simulink model "vehicle_hostmodel_2022b_v10"  (R2024b)
settings: Solver=ode4  StartTime=0.0  StopTime=inf  FixedStep=0.01  MaxStep=0.05  RelTol=1e-3
PreLoadFcn:
  | load("FInalGraph.mat")
model workspace (MAT data in the model file):
  G_final : digraph (value not decoded)
values from neighbouring files (symbols this model uses):
  ActorID = 0    [HelperSpeedActionAdapter.m]
  D = cross(B-A,C-A)    [HelperCalculateEgoRefPathInfo.m]
  L = zeros(N,1)    [HelperCalculateEgoRefPathInfo.m]
  psi_o = -1.185    [sensor.m]
  R = NaN(N,1)    [HelperCalculateEgoRefPathInfo.m]
  SceneInfo = [-32.1351766513 25.1612903226 -74.2242703533 -71.4592933948 -32.2887864823 26.2365591398 26.8509984639 27.0046082949 -32.7496159754 -72.380952381 -49.846390169 -49.3855606759 ... (30 elements, 10x3)]    [SceneLabels.mat]
  Ts = 0.05    [sensor.m]
undefined symbols (not defined in the file or in its folder): Acceleration, AngularVelocity, barrier_1, barrier_2, barrier_3, curvature, DefaultGear, DEND_B, DEND_S, DEND_T, direction, DiscIntNeverNeededParam, driving, finalint, goal1_coordinates, goal2_coordinates, goal3_coordinates, gradbp, latlongcoordinates, LF, LR, matlabshared, MAX_BRAKE, MAX_STEER, MAX_TORQUE, MCAR, MIN_BRAKE, MIN_STEER, MIN_TORQUE, NUMD_B, NUMD_S, NUMD_T, Pitch, Position, Roll, RRdamp, session, sigbuilder_block, STEER_RATIO, stopSign_ID, Tdead, thetaRefs, TL_ID, TrackWidth, ts, Vdead, Velocity, WB, xRef2s, Yaw, yRef2s
libraries: simulink x12, drivingscenarioandsensors x8, simulink_extras x5, drivingvehiclecontroller x2, trackingutilitieslib x2, robotalgslib x1, mpcadaslib x1, slpidlib x1, drivinglib x1, mpclib x1, autolibshared x1, vehdynlibviscommon x1
(part 4 of 4)

== matlab function vehicle_hostmodel_2022b_v10/MATLAB Function ==
  data: ttc output; dist output; left output; right output; LL_avail output; RL_avail output; tend2stay output; ego input; act input; LaneBounds input; RoadSpeed input; ego_vel output; stay output; LL_Change output; RL_Change output; y_lane output; LCinProgress input
function [ttc,dist,left,right,LL_avail,RL_avail,tend2stay,ego_vel,stay,LL_Change,RL_Change,y_lane] = fcn(ego,act,LaneBounds,RoadSpeed, LCinProgress)                       


%% Major tasks to look into

% Check the performance while transitioning into another lane 
% Lane change output when the ego on extreme lanes.
% Develop code to handle lane changes on road curvatures
% Integrate with the trajectory generation and check the perfomance
% Convert the code to ego vehicle coordinates


%%
%define some parameters
r_c = 20; %range considered to MIOs
t_min =  2;

num_actors = length(act.Actors);
%num_lanes = length(LaneBounds.LaneBoundaries)-1;


%% Using sensor data 
% TracksNum = Tracking.NumTracks;
% 
% 
% for t = 1:TracksNum
%     ObjectID(t) = Tracking.Tracks(t).ObjectClassID;
%     TrackPos(:,t) = Tracking.Tracks(t).State(1:2:5);
%     TrackVel(:,t) = Tracking.Tracks(t).State(2:2:6);

%% ego position and  velocity magnitude
ego_pos = ego.Position;
ego_vel = ego.Velocity(1);  % velocity

%ttc: (array) : agent.relative position / abs(relative velocity)
ttc = zeros(1,num_actors);
left = zeros(1,num_actors);
right = zeros(1,num_actors);

dist =  zeros(1,num_actors);
tend2stay=1;

%%
y_lane = zeros(1,length(LaneBounds.LaneBoundaries))

for l=1:length(y_lane)
    y_lane(l)=LaneBounds.LaneBoundaries(l).Coordinates(end,2)
end

%%
for i= 1:num_actors

    % Grab actor positions and velocities
    actor_pos = act.Actors(i).Position;   
    actor_vel = act.Actors(i).Velocity(1);  % x-component velocity

    %relative velocity of the agent
    rel_vel = actor_vel - ego_vel;


    %% Check if the actor is within a r_c range. If it is out of range, pass lane change as '1' automatically.

   dist(i) = norm([actor_pos(1) actor_pos(2)]-[ego_pos(1) ego_pos(2)]);
        
    if dist(i) > r_c
        left(i)=1;
        right(i)=1;
        continue
    end

    %% Check if the actor is in the same lane as that of ego

    % If the actor and ego are in the same lane, it is considered a lead/following vehicle in the same lane and by defualt, the lane change flag is 1.

    if (actor_pos(2)< (ego_pos(2)+0.5) && actor_pos(2) > (ego_pos(2)-0.5))
        if (rel_vel < 0 && ego_vel < (RoadSpeed+5) && actor_pos(1) > ego_pos(1) )
            left(i) =1;
            right(i)=1;
            tend2stay=0;        % we need to incorporate too slow condition even when the relative velocity is greater than 0.

        elseif (rel_vel < 0 && ego_vel < (RoadSpeed+5) && actor_pos(1) < ego_pos(1) )
            left(i) =1;
            right(i)=1;
            tend2stay=1;
        end

        continue
    end

    
    %% calculate ttc for the rest of the vehicles


    ttc(i) = (actor_pos(1)-ego_pos(1))/abs(rel_vel);

    % checking conditions for other surrounding actors

    % all actors on the left lane of the ego vehicle
%%
    if actor_pos(2)-ego_pos(2) > 0  

        if and(rel_vel>0, ttc(i) > t_min)  % target vehicles on the front of ego vehicle (any lane)
    
            left(i)=1; 
            right(i)=1;
    
        elseif (ttc(i)<0 && rel_vel<0 && abs(ttc(i)) > t_min)    % target vehicle on the back of ego vehicle (ttc<0) (any lane)
            left(i) =1;
            right(i)=1;
    
        else 
            left(i) =0;
            right(i)=1;
    
        end

    % all actors on the right lane of the ego vehicle

    elseif actor_pos(2)-ego_pos(2) < 0
         
        if and(rel_vel>0, ttc(i) > t_min)  % target vehicles on the front of ego vehicle (any lane)
    
            left(i)=1;
            right(i)=1;
    
        elseif (ttc(i)<0 && rel_vel<0 && abs(ttc(i)) > t_min)    % target vehicle on the back of ego vehicle (ttc<0) (any lane)
            left(i) =1;
            right(i)=1;
    
        else 
            left(i) =1;
            right(i)=0;
    
        end
    end
%%

end

%% check if the vehicle is in the extreme end lanes

    if ego_pos(2)<y_lane(1) && ego_pos(2)>y_lane(2)

        LL=0; RL=1;
    elseif ego_pos(2) > y_lane(end) && ego_pos(2) < y_lane(end-1)
        RL=0; LL=1;
    else 

        RL=1;LL=1;
    end

%%
LL_avail = all(left) %&& LL;

RL_avail = all(right) %&& RL               %&& ~lcLeft ; this can be decided later 


%% final commands

stay = tend2stay || ~(tend2stay || LL_avail || RL_avail);
LL_Change =  ~tend2stay && LL_avail ;

RL_Change =  ~tend2stay && RL_avail && ~LL_Change ;
LCFlag = ~stay;
if LCFlag && LCinProgress
    LCFlag = false;
    stay = ~LCFlag;
end

%% 






end

== matlab function vehicle_hostmodel_2022b_v10/Vehicle Dynamics/Info2ActorState/MATLAB Function2 ==
  data: aX input; Acceleration output; aY input; aZ input
function Acceleration = fcn(aX, aY, aZ)

Acceleration = [aX aY, aZ];

== matlab function vehicle_hostmodel_2022b_v10/Vehicle Dynamics/Info2ActorState/MATLAB Function3 ==
  data: phiDot input; AngularVelocity output; thetaDot input; psiDot input
function AngularVelocity = fcn(phiDot, thetaDot, psiDot)

AngularVelocity = [phiDot thetaDot, psiDot];

== stateflow chart vehicle_hostmodel_2022b_v10/Vehicle Dynamics/VehicleDynamics/engine-steer-brake dynamics/GearSelection1 ==
  state Park
    CurrGear = 0;
  state Reverse
    CurrGear = -1;
  state drive
    CurrGear = 1;
  (default) -> (junction 12)
  (junction 12) -> Reverse [order 3] : [DefaultGear == -1]
  (junction 12) -> drive [order 2] : [DefaultGear == 1]
  (junction 12) -> Park [order 1] : [DefaultGear == 0]
  (junction 12) -> Park [order 4] : %fallback to park
  drive -> Park [order 2] : [gear_cmd == 0 && allowShift(vc,Tbrake)]
  Park -> Reverse [order 2] : [gear_cmd == -1 && allowShift(vc,Tbrake)]
  Park -> drive [order 1] : [gear_cmd == 1 && allowShift(vc,Tbrake)]
  Reverse -> Park [order 2] : [gear_cmd == 0 && allowShift(vc,Tbrake)]
  drive -> Reverse [order 1] : [gear_cmd == -1 && allowShift(vc,Tbrake)]
  Reverse -> drive [order 1] : [gear_cmd == 1 && allowShift(vc,Tbrake)]
  data: Tdead parameter; Vdead parameter; vel function_input; brakeT function_input; allow function_output; CurrGear output; Tbrake input; vc input; gear_cmd input; DefaultGear parameter
  function allow = allowShift(vel, brakeT):
    | function allow = allowShift(vel, brakeT)
    | allow = (abs(vel) <= Vdead) && (abs(brakeT)>Tdead);
    | end

== matlab function vehicle_hostmodel_2022b_v10/Vehicle Dynamics/VehicleDynamics/engine-steer-brake dynamics/compute net torque ==
  data: gear input; Tnet output; Tengine input; Tbrake input; vc input
function Tnet  = net_torque(gear,Tengine,Tbrake,vc)

%  --set engine torque based on current gear selection

if (gear == 0)
    %  --vehicle is in PARK, so force engine torque to zero
    Tengine = 0;
end

Tnet = Tengine + Tbrake*tanh(5*vc);

end

== matlab function vehicle_hostmodel_2022b_v10/Vehicle Dynamics/VehicleDynamics/engine-steer-brake dynamics/gear selection state machine ==
  data: gear output; gear_cmd input; vc input; Tbrake input; Tdead input; Vdead input
function gear = gear_change_FSM(gear_cmd,vc,Tbrake,Tdead,Vdead)

persistent GEAR

%  The vehicle gear can take on one of the following enumerated values:
%  -1 = REVERSE
%   0 = PARK
%   1 = DRIVE

%  --initialize the local persistent variables

if isempty(GEAR)
    %  --default gear at startup is PARK
    %  Note:  Change this to 1 if you want car to initialize in DRIVE
    GEAR = 0;
end


%  --evaluate the gear change finite state machine

switch GEAR
    case 0  % vehicle is in PARK
        if (gear_cmd == 1)
            %  --check to see if we can shift to DRIVE
            if ((abs(vc) <= Vdead) && (abs(Tbrake) > Tdead))
                %  --shift to DRIVE
                GEAR = 1;
            end
            
        elseif (gear_cmd == 2)
            %  --check to see if we can shift to REVERSE
            if ((abs(vc) <= Vdead) && (abs(Tbrake) > Tdead))
                %  --shift to REVERSE
                GEAR = 2;
            end
        end
        
    case 1  % vehicle is in DRIVE
        if (gear_cmd == 0)
            %  --check to see if we can shift to PARK
            if ((abs(vc) <= Vdead) && (abs(Tbrake) > Tdead))
                %  --shift to PARK
                GEAR = 0;
            end
            
        elseif (gear_cmd == 2)
            %  --check to see if we can shift to REVERSE
            if ((abs(vc) <= Vdead) && (abs(Tbrake) > Tdead))
                %  --shift to REVERSE
                GEAR = 2;
            end
        end
        
    case -1  % vehicle is in REVERSE
        if (gear_cmd == 0)
            %  --check to see if we can shift to PARK
            if ((abs(vc) <= Vdead) && (abs(Tbrake) > Tdead))
                %  --shift to PARK
                GEAR = 0;
            end
            
        elseif (gear_cmd == 1)
            %  --check to see if we can shift to DRIVE
            if ((abs(vc) <= Vdead) && (abs(Tbrake) > Tdead))
                %  --shift to DRIVE
                GEAR = 1;
            end
        end
        
    otherwise  %  --should never be here
        if (vc > Vdead)
            %  --moving forward, so must be in DRIVE
            GEAR = 1;
        elseif (vc < -Vdead)
            %  --moving backward, so must be in REVERSE
            GEAR = 2;
        else
            %  --vehicle stoppped, so must be in PARK
            GEAR = 0;
        end

end


%  --output the current actual gear setting

gear = GEAR;

return

== matlab function vehicle_hostmodel_2022b_v10/Subsystem2/MATLAB Function5 ==
  data: OutWP output; NWP input; Flag input; WP input; CheckPointFlag input; PrevCF input
function OutWP   = OutputWP(NWP,Flag,WP,CheckPointFlag,PrevCF)

OutWP = zeros(600,2);

if Flag == 0 || (PrevCF ~= CheckPointFlag) 
    OutWP = WP(:,1:2);
else
    OutWP = NWP;
end

end

== stateflow chart vehicle_hostmodel_2022b_v10/Behavioural Planner/Chart ==
  settings: updateMethod=DISCRETE  sampleTime=Ts
  state Stationary
    en,du:
    VelCmd = 0;
    CurrentVelCmd = VelCmd;
    Navi = 0;
    Trans = 0;
    StopSim = 0;
    Tgap = 1;
  state Navigation
    state RailCrossing
      state Stop
        en:
        VelCmd = 0;
        Braking = 1;
        CurrentVelCmd = VelCmd;
      state Approaching
        en:
        Braking = 1;
        Tgap = 0;
        Trans = 0;
      state Transition
        en:
        Tgap = 1;
        Trans = 1;
        Braking = 0;
        VelCmd = SceneSpeed;
        CurrentVelCmd = VelCmd;
      state ExitScene
        en:
        ExitFlag = 1;
      (default) -> Navigation.RailCrossing.Approaching
      Navigation.RailCrossing.Approaching -> Navigation.RailCrossing.Stop [order 1] : [D2S <= 6 && (RRCross == 1 || ObjectDist <= TransDist)]
      Navigation.RailCrossing.Transition -> Navigation.RailCrossing.Approaching [order 2] : [ObjectDist <= TransDist]
      Navigation.RailCrossing.Approaching -> Navigation.RailCrossing.Transition [order 3] : [RRCross == 0 && ObjectDist > TransDist && D2S <= 6]
      Navigation.RailCrossing.Stop -> Navigation.RailCrossing.Transition : [RRCross == 0 && ObjectDist > TransDist]
      Navigation.RailCrossing.Approaching -> Navigation.RailCrossing.ExitScene [order 2] : [SceneID ~= 10]
      Navigation.RailCrossing.Transition -> Navigation.RailCrossing.ExitScene [order 1] : [SceneID == 0]
    state RoundAbout
      state Approaching
        en:
        Braking = 1;
        Trans = 0;
        Tgap = 0;
      state Stop
        en:
        VelCmd = 0;
        Braking = 1;
        CurrentVelCmd = VelCmd;
      state ExitScene
        en:
        ExitFlag = 1;
      state Transition
        en:
        Tgap = 1;
        Trans = 1;
        Braking = 0;
        VelCmd = SceneSpeed;
        CurrentVelCmd = VelCmd;
      (default) -> Navigation.RoundAbout.Approaching
      Navigation.RoundAbout.Approaching -> Navigation.RoundAbout.Stop [order 1] : [D2S <= 6]
      Navigation.RoundAbout.Stop -> Navigation.RoundAbout.Transition : [Clear2Go == 1]
      Navigation.RoundAbout.Approaching -> Navigation.RoundAbout.ExitScene [order 2] : [SceneID ~= 9]
      Navigation.RoundAbout.Transition -> Navigation.RoundAbout.ExitScene : [SceneID == 0]
    state DestCheck
      en,du:
      % dest reached?
      (default) -> (junction 47)
      (junction 47) -> (junction 48) [order 1] : [D2D < 2]
      (junction 47) -> (junction 49) [order 2] : {DestReached = 0;}
      (junction 48) -> (junction 50) : {DestReached = 1;}
      (junction 50) -> (junction 49) : {StopSim = 1;}
      (junction 49) -> (junction 51)
    state TrafficLight
      note: Yellow light duration is 1s
      state Stop
        en:
        Braking = 1;
        VelCmd = 0;
        CurrentVelCmd = VelCmd;
      state Approaching
        en:
        Tgap = 0;
        Trans = 0;
        T2S = 0;
        %if TLstate(1,4) == 1
        Braking = 1;
        %else
        % ACC = 0;
        %end
      state DecisionOnYellow
        en:
        T2S = D2S/EgoSpeed;
      state Transition
        en:
        Trans = 1;
        Braking = 0;
        Tgap = 1;
        VelCmd = SceneSpeed;
        CurrentVelCmd = VelCmd;
      state ExitScene
        en:
        ExitFlag = 1;
      DecisionOnYellow -> Navigation.TrafficLight.Approaching [order 1] : [T2S > 1.2]
      (default) -> Navigation.TrafficLight.Approaching
      Navigation.TrafficLight.Approaching -> Navigation.TrafficLight.Stop [order 1] : [D2S <= 6]
      Navigation.TrafficLight.Stop -> Navigation.TrafficLight.Transition : [TLstate(1,4) == 3 && ObjectDist > TransDist]
      Navigation.TrafficLight.Transition -> Navigation.TrafficLight.Approaching [order 2] : [TLstate(1,4) == 1  || ObjectDist < TransDist]
      Navigation.TrafficLight.Approaching -> Navigation.TrafficLight.Transition [order 2] : [TLstate(1,4) == 3 && ObjectDist > TransDist]
      Navigation.TrafficLight.Approaching -> Navigation.TrafficLight.ExitScene [order 3] : [SceneID ~= 8]
      Navigation.TrafficLight.Transition -> DecisionOnYellow [order 3] : [TLstate(1,4) == 2]
      DecisionOnYellow -> Navigation.TrafficLight.Transition [order 2] : [T2S <= 1.2]
      Navigation.TrafficLight.Transition -> Navigation.TrafficLight.ExitScene [order 1] : [SceneID == 0]
    state SceneRecognition
      en :
      VelCmd = RoadSpeed;
      CurrentVelCmd = VelCmd;
      ExitFlag = 0;
    state Go
      en:
      VelCmd = RoadSpeed;
      CurrentVelCmd = VelCmd;
      Trans = 0;
      ExitFlag = 0;
      Braking = 0;
    state StopSign
      state Approaching
        en:
        Braking = 1;
        Trans = 0;
        Tgap = 0;
      state Stop
        en:
        VelCmd = 0;
        Braking = 1;
        CurrentVelCmd = VelCmd;
      state ExitScene
        en:
        ExitFlag = 1;
      state Transition
        en:
        Trans = 1;
        Braking = 0;
        Tgap = 1;
        VelCmd = SceneSpeed;
        CurrentVelCmd = VelCmd;
      (default) -> Navigation.StopSign.Approaching
      Navigation.StopSign.Approaching -> Navigation.StopSign.Stop [order 1] : [D2S <= 7]
      Navigation.StopSign.Stop -> Navigation.StopSign.Transition : [after(3,sec) && Clear2Go == 1]
      Navigation.StopSign.Approaching -> Navigation.StopSign.ExitScene [order 2] : [SceneID ~= 7]
      Navigation.StopSign.Transition -> Navigation.StopSign.ExitScene : [SceneID == 0]
    Go -> RailCrossing [order 2] : [SceneID == 10]
    SceneRecognition -> RailCrossing [order 1] : [SceneID == 10]
    RailCrossing -> Go : [ExitFlag == 1]
    Go -> RoundAbout [order 3] : [SceneID == 9]
    SceneRecognition -> RoundAbout [order 2] : [SceneID == 9]
    RoundAbout -> Go : [ExitFlag == 1]
    (default) -> DestCheck
    SceneRecognition -> TrafficLight [order 4] : [SceneID == 8]
    DestCheck -> SceneRecognition : [DestReached == 0]
    Go -> TrafficLight [order 4] : [SceneID == 8]
    SceneRecognition -> DestCheck [order 5] : [D2D < 2]
    SceneRecognition -> StopSign [order 3] : [SceneID == 7]
    TrafficLight -> Go : [ExitFlag == 1]
    StopSign -> Go : [ExitFlag == 1]
    Go -> DestCheck [order 1] : [SceneID == 0]
    Go -> StopSign [order 5] : [SceneID == 7]
  (default) -> Stationary
  Stationary -> Navigation : [Navigate == 1]
  Navigation -> Stationary : [Navigate == 0 || DestReached == 1]
  data: TLstate input; TransDist input; ApproachingSpeed input; EgoSpeed input; ObjectDist input; SceneSpeed input; SDist input; RRCross input; D2S input; DestReached local; Navigate input; ExitFlag local; D2D input; Clear2Go input; RoadSpeed input; CurrentVelCmd local; Navi local; VelCmd output; SceneID input; Tgap output; Trans output; StopSim output; Braking output; T2S local

== matlab function vehicle_hostmodel_2022b_v10/Subsystem2/Subsystem1/MATLAB Function1 ==
  data: waypoints input; NewPoints output; current_point input; barrier input; CheckPointFlag input
function NewPoints = NOptPath(waypoints,current_point,barrier,CheckPointFlag)

coder.extrinsic("NewOptimalPath2");
NewPoints = zeros(600,2);
%Nx = [1];
%Ny = [1];
%coder.varsize('Nx','Ny')
NewPoints = NewOptimalPath2(waypoints,current_point,barrier,CheckPointFlag);
%NewPoints = [Nx,Ny]

end

== matlab function vehicle_hostmodel_2022b_v10/Subsystem/Function-Call Subsystem/MATLAB Function1 ==
  data: EgoPosition input; MIOPos input; curvature input; MIOVel input; V_i input; xd output; yd output; laneL input; laneR input; V_desired input; LCinProgress output
function [xd,yd,LCinProgress] = traj(EgoPosition,MIOPos,curvature,MIOVel, V_i, laneL, laneR, V_desired)
Vx_i =0;Vx_f=0;Vy_i=0;Vy_f=0;Ax_i=0;Ax_f=0;Ay_i=0;Ay_f=0;T_i=0;T_f=0;V_f=0;A_f=0;x_set=0;y_set=0;theta4=0;

P = zeros(6,6);
% xq = zeros(1,size(RefPath,1)); yq = zeros(1,size(RefPath,2));
EgoPosition(1,2)=-EgoPosition(1,2);
x_init= EgoPosition(1,1)+2; y_init = EgoPosition(1,2)-2;
% xq = RefPath(:,1)'; 
% yq = RefPath(:,2)';
num_foc_t = 98;
V_max= V_desired; ad_n=0; vd_n=MIOVel; wd_n=vd_n*curvature;
lane_width = 3.6 * (laneL-laneR); % +1 if left of current lane and -1 if right of current lane(rahul flipped)
xd = zeros(num_foc_t+1,1); 
yd = zeros(num_foc_t+1,1);
xf =0; 
yf = 0;

    %xf = [EgoPosition(1,1)+ MIOPos(1) ]; yf = [ EgoPosition(1,2)+ MIOPos(2) + lane_width];  
    xf = [EgoPosition(1,1)+ 20 ]; yf = [EgoPosition(1,2)+ lane_width]; % 80
    V_f = V_max;
    W_f = V_f*curvature;
    A_f = 0;

    %dist2crash = sqrt((x_init-MIOPos(1))^2+(y_init-MIOPos(2))^2);
    %dist2crash = 40;
    %T_f = abs(dist2crash/(MIOVel-V_i));
    T_f = 3;
    P = [1, T_i, T_i^2, T_i^3, T_i^4, T_i^5;
         0, 1, 2*T_i, 3*T_i^2, 4*T_i^3, 5*T_i^4;
         0, 0, 2, 6*T_i, 12*T_i^2, 20*T_i^3;
         1, T_f, T_f^2, T_f^3, T_f^4, T_f^5;
         0, 1, 2*T_f, 3*T_f^2, 4*T_f^3, 5*T_f^4;
         0, 0, 2, 6*T_f, 12*T_f^2, 20*T_f^3];

%     mtang4 = (yq(1,index+2)-yq(1,index+1))/(xq(1,index+2)-xq(1,index+1));

    Vx_i = vd_n*cos(theta4); 
    Vy_i = vd_n*sin(theta4); 
    Ax_i = ad_n*cos(theta4)-vd_n*sin(theta4)*wd_n; 
    Ay_i = ad_n*sin(theta4)+vd_n*cos(theta4)*wd_n;

%     if(xq(index+2)-xq(index+1)<0)
%         theta_4 = pi + atan(mtang4);
%     else
%         theta_4 = atan(mtang4);
%     end

    theta_4 =0;
    Vx_f = V_f*cos(theta_4); % curvature angle
    Vy_f = V_f*sin(theta_4);
    Ax_f = A_f*cos(theta_4)-V_f*sin(theta_4)*W_f;
    Ay_f = A_f*sin(theta_4)+V_f*cos(theta_4)*W_f;

    g1 = [x_init; Vx_i; Ax_i; xf; Vx_f; Ax_f];
    g2 = [y_init; Vy_i; Ay_i; yf; Vy_f; Ay_f];

    a_coeff = P\g1;
    b_coeff = P\g2;
    
    td = T_i;
    scatter(x_init,y_init,'go')
    hold on; 
    scatter(xf,yf,'ro')
    hold on;
    
    for f = 1:(num_foc_t+1)
        xd(f,1) = [1,td,td^2,td^3,td^4,td^5]*a_coeff 
        yd(f,1) = [1,td,td^2,td^3,td^4,td^5]*b_coeff
        td = td + (T_f - T_i)/num_foc_t;
        scatter(xd(f,1),yd(f,1),'y.');
    end

LCinProgress = 1;

% hold on;
end

== matlab function vehicle_hostmodel_2022b_v10/Subsystem2/MATLAB Function2 ==
  data: CurrentPose input; origin input; CurrPosLL output
function CurrPosLL =  LLAcoordinates(CurrentPose,origin)
xyzenu = [CurrentPose(1) CurrentPose(2) 0];
lla = enu2lla(xyzenu,origin,'ellipsoid');
CurrPosLL = [lla(1),lla(2)];

== matlab function vehicle_hostmodel_2022b_v10/Behavioural Planner/MATLAB Function1 ==
  data: EgoLength input; TransDist output; IntDist input
function TransDist = IntersectionClearanceDist(EgoLength,IntDist)

TransDist = IntDist + EgoLength;

== matlab function vehicle_hostmodel_2022b_v10/Subsystem/Turns LC in prog off ==
  data: u input; y output
function y = fcn(u)

persistent counter;
persistent input_high;

if isempty(counter)
    counter = 0;
end

if isempty(input_high)
    input_high = false;
end

if u ~= 0
    input_high = true;
end

if input_high && counter < 100
    y = u;
    counter = counter + 1;
else
    y = 0;
end

== matlab function vehicle_hostmodel_2022b_v10/MATLAB Function3 ==
  data: CurrentPose input; barrier1 input; barrier2 input; barrier3 input; ChkPointFlag input; FlagBarrier output; distanceBarrier input; outbarrier output; dist output
function [FlagBarrier, outbarrier,dist] =  BarrierFlag(CurrentPose,barrier1,barrier2,barrier3,ChkPointFlag,distanceBarrier)

outbarrier = barrier1;
if ChkPointFlag <1 
    dist = distance(CurrentPose(1),CurrentPose(2),barrier1(1),barrier1(2));
elseif ChkPointFlag>=1 && ChkPointFlag < 3
    outbarrier = barrier2;
    dist = distance(CurrentPose(1),CurrentPose(2),outbarrier(1),outbarrier(2));
else
    outbarrier = barrier3;
    dist = distance(CurrentPose(1),CurrentPose(2),outbarrier(1),outbarrier(2));
end

if dist>distanceBarrier
    FlagBarrier = 0;
else
    FlagBarrier = 1;
end

function d = distance(lat0,lon0,lat1,lon1)
    phi0 = lat0*(pi/180);
    phi1 = lat1*(pi/180);
    delta_lambda = (lon1-lon0)*(pi/180);
    d = 6371000*acos(sin(phi0)*sin(phi1)+cos(phi0)*cos(phi1)*cos(delta_lambda));
end

end

== matlab function vehicle_hostmodel_2022b_v10/MATLAB Function4 ==
  data: Waypoints input; WPENU output; origin input; height input; dest output; goalcoord input
function [WPENU,dest]  = ENUcoord(Waypoints,origin,height,goalcoord)
heights = height*ones(600,1);
Waypoints_h = cat(2,Waypoints,heights);
WPENU1 = zeros(600,3);
WPENU = zeros(600,2);
WPENU1 = lla2enu(Waypoints_h,origin,'ellipsoid');
destination = zeros(1,3);
dest = zeros(1,2);
goal = cat(2,goalcoord,height);
destination = lla2enu(goal,origin,'ellipsoid');
dest = [destination(1),destination(2)];
WPENU = WPENU1(:,1:2);

== matlab function vehicle_hostmodel_2022b_v10/Subsystem2/MATLAB Function6 ==
  data: BarrierFlag input; Flag output; Flag input; PrevFlag input; trigger output
function [Flag,trigger] = Switch(BarrierFlag,Flag, PrevFlag)

if BarrierFlag
    Flag = Flag + BarrierFlag;
end

if Flag ~= PrevFlag
    trigger = 1;
else
    trigger = 0;
end

end

== matlab function vehicle_hostmodel_2022b_v10/Behavioural Planner/MATLAB Function2 ==
  data: Dest input; D2D output; CurrentPose input
function D2D = fcn(Dest, CurrentPose)
%CurrentPose(2) = -CurrentPose(2);
%D2D = norm(Dest - CurrentPose(1:2)');

D2D=sqrt((CurrentPose(1)-Dest(1,1))^2+(CurrentPose(2)-Dest(1,2))^2);
end

== matlab function vehicle_hostmodel_2022b_v10/Subsystem/PathPlanner/MATLAB Function3 ==
  settings: updateMethod=DISCRETE
  data: out output; check output; Xref input; Yref input; xd input; yd input; LC input; current_pos input; d2f input; dcheck output
function [out,check,dcheck]  = PathPlanning(Xref, Yref, xd, yd, LC, current_pos, d2f)

persistent output_matrix
persistent lc_triggered

if isempty(lc_triggered)
lc_triggered = false;
end

%lc_triggered=0;
%if isempty(hold_output)
  %  hold_output = false;
%end


if isempty(output_matrix)
    output_matrix = [Xref(:), Yref(:)];
    out = [Xref(:), Yref(:)];
else
    out = output_matrix;
end

if LC && ~isempty(xd) && ~isempty(yd)
    output_matrix = [xd(:), yd(:)];
    lc_triggered=true;
       
end

check=lc_triggered;
dcheck=output_matrix;
%out=output_matrix;

if lc_triggered && d2f < 5 %&& ~isempty(output_matrix) %&& ~hold_output
    %Yout = Yref(:);
    if current_pos > 0
        Xout = Xref(:);
        Yout = Yref + 3.6;
    else
        Xout = Xref(:);
        Yout = Yref;
    end
    output_matrix = [Xout, Yout];
    out=output_matrix;
    lc_triggered=false;
    %hold_output = true;
end

out=output_matrix;




%if ~LC && ~isempty(output_matrix) && lc_triggered
    %hold_output = false;
    %lc_triggered=false;
%end

end

== stateflow chart vehicle_hostmodel_2022b_v10/Behavioural Planner/Routing ==
  state InitialRoute
    en:
    NewRoute = 0;
  state Rerouting
    en:
    NewRoute = 1;
  (default) -> InitialRoute
  InitialRoute -> Rerouting : [ReRoute == 1]
  Rerouting -> InitialRoute : [ReRoute == 0]
  data: ReRoute input; NewRoute output

== matlab function vehicle_hostmodel_2022b_v10/Controllers/Lateral Controllers1/Pure Pursuit Controller1/MATLAB Function ==
  data: ld input; e output; alpha input; L input
function e = cte(ld,alpha,L)
K = 2*sin(alpha)/ld;
e = (K*ld^2)/2;

== matlab function vehicle_hostmodel_2022b_v10/Subsystem2/MATLAB Function1 ==
  data: curr_point input; CheckPointFlag output; checkpoint input; dist output; checkpoint1 input; Prev_Flag input; trigger output; CheckPointFlag input
function [CheckPointFlag,dist,trigger]= ChkPointFlag(curr_point,checkpoint,checkpoint1,Prev_Flag,CheckPointFlag)

if CheckPointFlag ~= Prev_Flag
    checkpoint2 = checkpoint1;
else
    checkpoint2 = checkpoint;
end

dist = distance(curr_point(1),curr_point(2),checkpoint2(1),checkpoint2(2));

if dist < 1 && CheckPointFlag ~= Prev_Flag
    CheckPointFlag = CheckPointFlag + 1;
elseif dist < 1 && CheckPointFlag == Prev_Flag
    CheckPointFlag = CheckPointFlag;
elseif dist > 1
    CheckPointFlag = 0;
else
    CheckPointFlag = 0;
end

if CheckPointFlag ~= Prev_Flag
    trigger = 1;
else
    trigger = 0;
end

function d = distance(lat0,lon0,lat1,lon1)
    phi0 = lat0*(pi/180);
    phi1 = lat1*(pi/180);
    delta_lambda = (lon1-lon0)*(pi/180);
    d = 6371000*acos(sin(phi0)*sin(phi1)+cos(phi0)*cos(phi1)*cos(delta_lambda));
end
end

== matlab function vehicle_hostmodel_2022b_v10/Subsystem2/MATLAB Function7 ==
  data: WP input; OWP output; CheckPointFlag input
function OWP = TrajectoryPoints(WP,CheckPointFlag)

OWP = zeros(600,3);

extra_idx = 10;

op1 = 199;
op2 = 100;
op3 = 87;

if CheckPointFlag < 1
    for i = 1:(op1+extra_idx)
        OWP(i,:) = WP(i,:);
    end
    for j = 1:length(OWP)
        if OWP(j,:) == [0,0,0]
            OWP(j,:) = WP(op1,:);
        end
    end
elseif CheckPointFlag >= 1 && CheckPointFlag < 3
    for k = 1:(op2+extra_idx)
        OWP(k,:) = WP(k+op1,:);
    end
    for l = 1:length(OWP)
        if OWP(l,:) == [0,0,0]
            OWP(l,:) = WP(op1+op2,:);
        end
    end
else
    for m = 1:op3
        OWP(m,:) = WP(m+op2+op1,:);
    end
    for n = 1:length(OWP)
        if OWP(n,:) == [0,0,0]
            OWP(n,:) = WP(op1+op2+op3,:);
        end
    end
end
end

== matlab function vehicle_hostmodel_2022b_v10/Subsystem2/MATLAB Function8 ==
  data: flag input; flag output; checkpointflag input; checkpointarray input; checkpointarray output
function [flag,checkpointarray]= CFlag(flag,checkpointflag,checkpointarray)


if checkpointflag == 1 && checkpointarray(1) < 1 && checkpointarray(2) < 1
    flag = flag + checkpointflag;
    checkpointarray(1) = 1;
elseif checkpointflag == 1 && checkpointarray(1)>=1 && checkpointarray(2)<1
    flag = flag+checkpointflag;
    checkpointarray(2) = 1;
elseif checkpointflag == 1 && checkpointarray(1)>=1 && checkpointarray(2)>=1
    flag = flag;
else
    flag = flag;
end
end

== matlab function vehicle_hostmodel_2022b_v10/MATLAB Function1 ==
  data: EgoWayPts input; IntWP output
function IntWP  = InterBlock(EgoWayPts)

IntWP = zeros(1000,2);

x1 = unique(EgoWayPts(:,1),'stable');
y1 = unique(EgoWayPts(:,2),'stable');

EGWP = [x1,y1];

distancematrix = squareform(pdist(EGWP));
distancesteps = zeros(length(EGWP)-1,1);
for i = 2:length(EGWP)
    distancesteps(i-1,1) = distancematrix(i,i-1);
end
totalDistance = sum(distancesteps); 
distbp = cumsum([0; distancesteps]); 
gradbp = linspace(0,totalDistance,1000);

% linearize X and Y vectors based on distance
xRef2 = interp1(distbp,x1',gradbp,'spline');
yRef2 = interp1(distbp,y1',gradbp,'spline');
% yRef2s = smooth(gradbp,yRef2); % smooth waypoints
% xRef2s = smooth(gradbp,xRef2); % smooth waypoints
IntWP = [xRef2',yRef2'];

== matlab function vehicle_hostmodel_2022b_v10/Controllers/MATLAB Function ==
  data: RefPoses input; y output; CurrPose input; CurrVel input; data output
function [y,data] = MPC(RefPoses,CurrPose,CurrVel)

%%lateral control 

%vehicle_parameters

tire_radius = 3.5;

N = 10; %horizon duration







y = u;

== matlab function vehicle_hostmodel_2022b_v10/MATLAB Function2 ==
  data: x_path input; ref_traj output; y_path input; curvature input; v_max input; current_position input; PredictionHorizon input; distances output
function [ref_traj, distances] = computeReferenceTrajectory(x_path, y_path, curvature, v_max, current_position, PredictionHorizon)
% This function computes the reference trajectory for lane following
% including x, y, yaw, longitudinal velocity (vx), lateral velocity (vy), and yaw rate (w).

    N = length(x_path);
    ref_traj = zeros(10, 6);

    % Find the closest point to the current position
    distances = sqrt((x_path - current_position(1)).^2 + (y_path - current_position(2)).^2);
    [~, closest_idx] = min(distances);

    % Select reference points starting from the closest waypoint
    start_idx = closest_idx;
    end_idx = min(N, start_idx + PredictionHorizon - 1);
    selected_indices = start_idx:end_idx;

    ref_traj(1:length(selected_indices), 1) = x_path(selected_indices);  % x_ref
    ref_traj(1:length(selected_indices), 2) = y_path(selected_indices);  % y_ref

    for i = 1:length(selected_indices)
        if abs(curvature(selected_indices(i))) <= 1e-2
            v_ref = v_max;  
        else
            r = 1 / abs(curvature(selected_indices(i))); 
            v_ref = min(v_max, sqrt(9.81 * r * 0.2));  
        end

        ref_traj(i, 4) = v_ref;  % vx_ref

        if i < length(selected_indices)
            dx = x_path(selected_indices(i+1)) - x_path(selected_indices(i));
            dy = y_path(selected_indices(i+1)) - y_path(selected_indices(i));
            yaw_ref = atan2(dy, dx);  
        else
            yaw_ref = ref_traj(i-1, 3);
        end
        ref_traj(i, 3) = yaw_ref;  % yaw_ref
        ref_traj(i, 5) = 0;  % vy_ref is zero to avoid lateral acceleration
        ref_traj(i, 6) = v_ref * curvature(selected_indices(i));  % w_ref = v * curvature
    end
end

== matlab function vehicle_hostmodel_2022b_v10/MATLAB Function5 ==
  data: vx input; throttle output; vy input; yaw input; yaw_rate input; x input; y input; refTraj input; steer output
function [throttle,steer] = SimMPC(vx,vy,yaw,yaw_rate,x,y,refTraj)

coder.extrinsic('MPC1');
throttle = zeros(1,1);
steer = zeros(1,1);
[throttle, steer] = MPC1(x, y, yaw, vx, vy, yaw_rate, refTraj);
end

== matlab function vehicle_hostmodel_2022b_v10/MATLAB Function6 ==
  data: u input; accel output; deccel output
function [accel, deccel] = computeAccelDeccel(u)
    if u > 0
        accel = u;    
        deccel = 0;  
    else
        accel = 0;   
        deccel = -u;  
    end
end

== matlab function vehicle_hostmodel_2022b_v10/MATLAB Function7 ==
  data: u input; throttle output; steer output
function [throttle, steer] = Command(u)

throttle = u(1);
steer = u(2);
end

== matlab function vehicle_hostmodel_2022b_v10/Controllers/Subsystem2/MATLAB Function ==
  data: u input; accel output; decel output
function [accel, decel] = fcn(u)
if(u>0)
    accel=u; decel=0;
elseif(u<0)
    accel=0; decel=-u;
else
    accel=0;decel=0;
end

== matlab function vehicle_hostmodel_2022b_v10/Controllers/Subsystem2/Subsystem/Desired Velocity Profile ==
  data: CurrVel input; DesiredDecel output; RelDist input
function DesiredDecel = VelocityProfile(CurrVel,RelDist)
% time remaining = (current velocity) / (deceleration).
% desired velocity = (stopping distance - current distance) / time remaining.
Dist = RelDist - (2.6850+2);
if RelDist <= 1*(2.6850+3)
    DesiredDecel = 10;
else
%     Dist = RelDist - (2.6850 + 3);
%     Decel = (CurrVel^2)/(2*Dist);
%     RemainingTime = CurrVel/Decel;
%     DesiredVel = Dist/RemainingTime; % DesiredVel = CurrVel/2
    Decel = (CurrVel^2)/(2*Dist);
    DesiredDecel = Decel;
end

== matlab function vehicle_hostmodel_2022b_v10/Controllers/Subsystem2/Subsystem/Function-Call Subsystem/MATLAB Function1 ==
  data: Vel input; BrakingAcc output; RelDist input
function BrakingAcc = fcn(Vel,RelDist)

DistOffset = 1;
Dist = RelDist - DistOffset;
BrakingAcc = (Vel^2)/(2*Dist);
